simulink model "inverted_pendulum"  (R2013a)
settings: Solver=ode45  StartTime=0.0  StopTime=10.0  RelTol=1e-3
values from neighbouring files (symbols this model uses):
  l = traj(size(traj,1),size(traj,2))    [f.m]    (also in findGradient2.m = 5; findGradientPend.m = 5; optimize.m = 5; rungd.m = 10)
  m = size(t,2)    [ff.m]    (also in findGradientPend.m; interpolate.m = min(dss,[],2))
undefined symbols (not defined in the file or in its folder): b, g, I, M
settings Model: Creator=simplehands  LastModifiedBy=simplehands

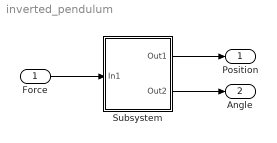
== system inverted_pendulum ==
  Force : Inport
  Subsystem : Subsystem
  Position : Outport
  Angle : Outport  Port=2
  wires:
  Force/1 -> Subsystem/1(In1)
  Subsystem/1(Out1) -> Position/1
  Subsystem/2(Out2) -> Angle/1

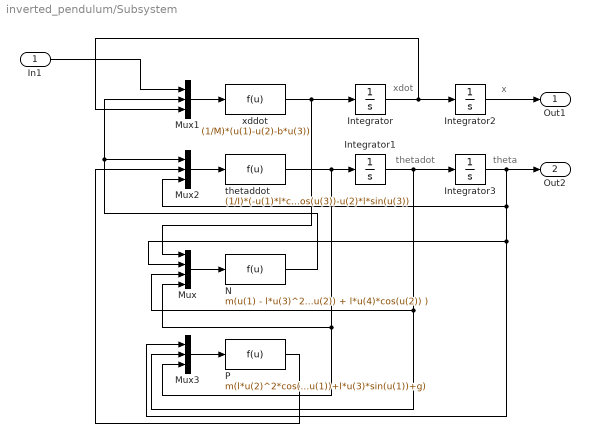
== system inverted_pendulum/Subsystem ==
  note: theta
  note: x
  note: thetadot
  note: xdot
  In1 : Inport
  Integrator : Integrator  ContinuousStateAttributes='x'
  Integrator1 : Integrator  ContinuousStateAttributes='theta'
  Integrator2 : Integrator  ContinuousStateAttributes='x'
  Integrator3 : Integrator  InitialCondition=pi  ContinuousStateAttributes='theta'
  Mux : Mux
  Mux1 : Mux  Inputs=3
  Mux2 : Mux  Inputs=3
  Mux3 : Mux  Inputs=3
  N : Fcn  Expr=m(u(1) - l*u(3)^2*sin(u(2)) + l*u(4)*cos(u(2)) )
  P : Fcn  Expr=m(l*u(2)^2*cos(u(1))+l*u(3)*sin(u(1))+g)
  thetaddot : Fcn  Expr=(1/I)*(-u(1)*l*cos(u(3))-u(2)*l*sin(u(3))
  xddot : Fcn  Expr=(1/M)*(u(1)-u(2)-b*u(3))
  Out1 : Outport
  Out2 : Outport  Port=2
  wires:
  Mux1/1 -> xddot/1
  Integrator3/1 -> Out2/1, Mux3/1, Mux/2, Mux2/3
  Integrator2/1 -> Out1/1
  Integrator/1 -> Mux1/3, Integrator2/1
  Integrator1/1 -> Mux/3, Mux3/2, Integrator3/1
  P/1 -> Mux2/2
  xddot/1 -> Mux/1, Integrator/1
  In1/1 -> Mux1/1
  thetaddot/1 -> Mux/4, Mux3/3, Integrator1/1
  Mux/1 -> N/1
  N/1 -> Mux2/1, Mux1/2
  Mux3/1 -> P/1
  Mux2/1 -> thetaddot/1
